simulink model "test"  (Simulink 7.4)
settings: Solver=ode5  SolverMode=SingleTasking  StartTime=0.0  StopTime=100.0  FixedStep=0.001  RelTol=1e-3
undefined symbols (not defined in the file): National_Instruments, PCI, St
libraries: rtwinlib x2
settings Model: Creator=mlab  LastModifiedBy=mlab  SimulationMode=external
settings HardwareCC: ProdIntDivRoundTo=Zero  ProdEndianess=LittleEndian  ProdHWDeviceType=Generic->32-bit x86 compatible
settings RTWCC: SystemTargetFile=rtwin.tlc  TemplateMakefile=rtwin.tmf  Description=Real-Time Windows Target  ProcessScript=rtwin_make_rtw_hook  RTWCompilerOptimization=On
settings CodeAppCC: MaxIdLength=95
settings RTWinTargetCC: TargetLibSuffix=_rtwin.lib  TargetPreCompLibLocation=C:\Program Files\MATLAB\R2009b\toolbox\rtw\targets\rtwin\lib  TargetFunctionLibrary=ANSI_C  PortableWordSizes=off

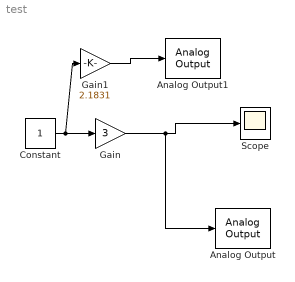
== system test ==
  Analog Output : rtwinlib/Analog Output  SampleTime=St  DrvName=National_Instruments/PCI-6229  DrvAddress=4294967295  DrvOptions=[0 0 0 0 0]  Channels=1  RangeMode=1  VoltRange=1  InitialValue=[]  FinalValue=[]
      settings: AttributesFormatString=National Instruments\nPCI-6229 [auto]
  Analog Output1 : rtwinlib/Analog Output  SampleTime=St  DrvName=National_Instruments/PCI-6229  DrvAddress=4294967295  DrvOptions=[0 0 0 0 0]  Channels=2  RangeMode=1  VoltRange=1  InitialValue=[]  FinalValue=[]
      settings: AttributesFormatString=National Instruments\nPCI-6229 [auto]
  Constant : Constant  OutDataType=fixdt(1, 16)  OutScaling=2^0
  Gain : Gain  Gain=3  ParameterDataType=fixdt(1, 16)  ParameterScaling=2^0  OutDataType=fixdt(1, 16)  OutScaling=2^0
  Gain1 : Gain  Gain=2.1831  ParameterDataType=fixdt(1, 16)  ParameterScaling=2^0  OutDataType=fixdt(1, 16)  OutScaling=2^0
  Scope : Scope
      settings: TickLabels=on  TimeRange=1  YMin=-1.5  YMax=1.5  SampleInput=on
  wires:
  Constant/1 -> Gain/1, Gain1/1
  Gain/1 -> Scope/1, Analog Output/1
  Gain1/1 -> Analog Output1/1
